simulink model "Test_controlled_3_phase_V_src_and_mut_induct"  (Simulink 7.7)
settings: Solver=ode45  StartTime=0.0  StopTime=10.0  RelTol=1e-3
libraries: powerlib x5, pm_machines_library x1
settings Model: Creator=s0237326  LastModifiedBy=s0237326

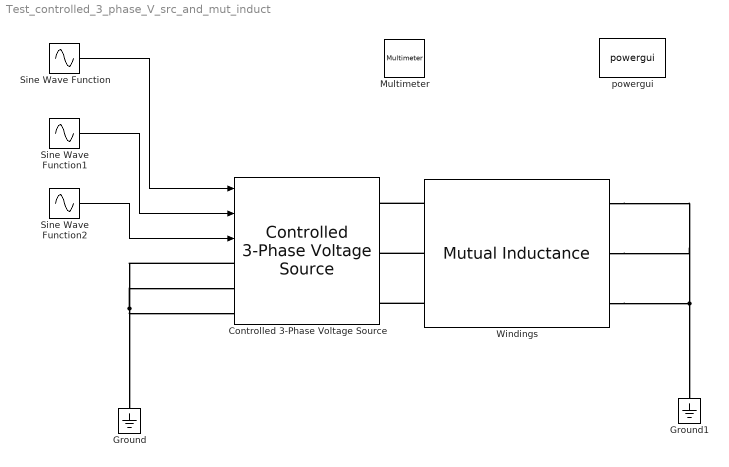
== system Test_controlled_3_phase_V_src_and_mut_induct ==
  Controlled 3-Phase Voltage Source : pm_machines_library/Controlled 3-Phase Voltage Source  SystemSampleTime=-1
      link override Controlled Voltage Source A: Source_Type=DC  Initialize=off
      link override Controlled Voltage Source C: Source_Type=DC  Initialize=off
      link override Controlled Voltage Source1: Source_Type=DC  Initialize=off
  Ground : powerlib/Elements/Ground  PhysicalDomain=powersysdomain  SubClassName=unknown  LeftPortType=p1  RightPortType=p1  LConnTagsString=a
  Ground1 : powerlib/Elements/Ground  PhysicalDomain=powersysdomain  SubClassName=unknown  LeftPortType=p1  RightPortType=p1  LConnTagsString=a
  Multimeter : powerlib/Measurements/Multimeter  SystemSampleTime=-1  PhasorSimulation=off  OutputType=Complex  sel=[1 4 2 5 3 6]  L=6  Gain=[1 1 1 1 1 1]  yselected={'Uw1: Windings','Iw1: Windings','Uw2: Windings','Iw2: Windings','Uw3: Windings','Iw3: Windings'};  PSBOutputType=1  PSBequivalent=0  AxesSetting=[0,0.1,-100,100]  Display=1  SavedBlockNames=-11
  Sine Wave Function : Sin  Frequency=6.28  SampleTime=0
  Sine Wave Function1 : Sin  Frequency=6.28  Phase=2.0944  SampleTime=0
  Sine Wave Function2 : Sin  Frequency=6.28  Phase=4.188  SampleTime=0
  Windings : powerlib/Elements/Mutual Inductance  PhysicalDomain=powersysdomain  SubClassName=unknown  LeftPortType=p1  RightPortType=p1  LConnTagsString=a|b|c  RConnTagsString=A|B|C  TypeOfMutual=Two or three windings with equal mutual terms  NumberOfWindings=3  SelfImpedance1=[44.03 0.3064]  SelfImpedance2=[44.03 0.3064]  ThreeWindings=on  SelfImpedance3=[44.03 0.3064]  MutualImpedance=[0 0.0119]  InductanceMatrix="[1.0 0.9  0.9 ;  0.9 1.0  0.9;  0.9 0.9 1.0 ] * 1e-3"  ResistanceMatrix="[1.0 0.9  0.9 ;  0.9 1.0  0.9;  0.9 0.9 1.0 ]"  Measurements=Winding voltages and currents
      settings: AttributesFormatString=\n
  powergui : powerlib/powergui  Priority=1  SystemSampleTime=-1  SimulationMode=Continuous  SampleTime=50e-6  frequency=60  SPID=off  DisableSnubberDevices=off  DisableRonSwitches=off  DisableVfSwitches=off  SwTol=0  Interpol=off  DisplayEquations=off  FunctionMessages=off  frequencyindice=0  Pbase=100e6  ErrMax=1e-4  Iterations=50  UnitsV=kV  UnitsW=MW  echomessages=off  HookPort=off  EnableUseOfTLC=off  x0status=blocks  RestoreLinks=warning  ResistiveCurrentMeasurement=off  Ylog=off  Xlog=on  ShowGrid=off  save=off  variable=ZData  ZoomFFT=off  StartTime=0.0  cycles=1  DisplayStyle=1  FreqAxis=off  MaxFrequency=1000  frequencyindicesteady=1  display=off  methode=off
  wires:
  Sine Wave Function/1 -> Controlled 3-Phase Voltage Source/1
  Sine Wave Function1/1 -> Controlled 3-Phase Voltage Source/2
  Sine Wave Function2/1 -> Controlled 3-Phase Voltage Source/3
  connections:
  Windings/LConn3 -- Controlled 3-Phase Voltage Source/RConn3
  Windings/LConn2 -- Controlled 3-Phase Voltage Source/RConn2
  Windings/LConn1 -- Controlled 3-Phase Voltage Source/RConn1
  Controlled 3-Phase Voltage Source/LConn1 -- Controlled 3-Phase Voltage Source/LConn2 -- Ground/LConn1 -- Controlled 3-Phase Voltage Source/LConn3
  Windings/RConn1 -- Windings/RConn2 -- Ground1/LConn1 -- Windings/RConn3
